simulink model "vehiclesim_mImplComplete"  (R2018a)
settings: Solver=FixedStepDiscrete  StartTime=0.0  StopTime=15  FixedStep=Ts  RelTol=1e-3  EnableMultiTasking=on
undefined symbols (not defined in the file): AL, Cd, cr1, cr2, fsw, g, i_t, Mv, p, rho_a, Rw, sigbuilder_block, Tmax, Ts, Tsi, V1, wbase
libraries: fl_lib x42, nesl_utility x16, pe_lib x5, pePwmGenerator x3, simulink x1
Description:
  | IPMSM Torque Control in an Axle-Drive EV
  | 
  | Copyright 2017 The MathWorks, Inc.
settings Model: Creator=The MathWorks, Inc.  LastModifiedBy=liamflaherty
settings SolverCC: AutoInsertRateTranBlk=on
settings DataIOCC: MaxDataPoints=510000  SignalLoggingName=logsout_pe_ipmsm_torque_control_ev_axle
settings OptimizationCC: LifeSpan=inf
settings DebuggingCC: UnderspecifiedInitializationDetection=Classic  MergeDetectMultiDrivingBlocksExec=none  SFUnexpectedBacktrackingDiag=warning  SFNoUnconditionalDefaultTransitionDiag=warning  SFExecutionAtInitializationDiag=none
settings CodeAppCC: StateflowObjectComments=on
settings GRTTargetCC: TargetLangStandard=C89/C90 (ANSI)  GeneratePreprocessorConditionals=Disable all
settings ConfigComp: CovMetricSettings=dw  CovHtmlReporting=on  CovSaveCumulativeToWorkspaceVar=on  CovSaveSingleToWorkspaceVar=on  CovExternalEMLEnable=off
settings SimscapeCC: SimscapeNormalizeSystem=off  SimscapeLogType=all  SimscapeLogSimulationStatistics=on  SimscapeLogName=simlog_pe_ipmsm_torque_control_ev_axle  SimscapeLogDataHistory=510000

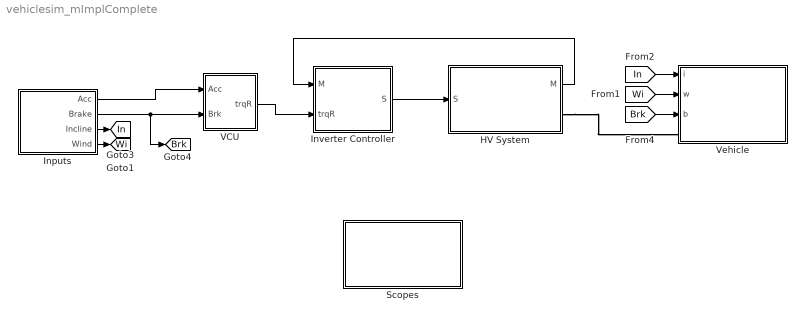
== system vehiclesim_mImplComplete ==
  HV System : Subsystem
  Inputs : Subsystem  Tag=STV Subsys  LoadFcn=sigbuilder_block('load');  StartFcn=sigbuilder_block('start');  StopFcn=sigbuilder_block('stop');  ClipboardFcn=sigbuilder_block('clipboard');  mask(Sigbuilder block){tuvar=[0:10]}
      mask help: Simulink:masks:SigbuilderBlock_MD
      mask init:
      | if ~strcmp(get_param(bdroot(gcbh),'SimulationStatus'),'stopped') tuvar = sigbuilder_block('maskInit'); end
      settings: CopyFcn=sigbuilder_block('copy');  DeleteFcn=sigbuilder_block('delete');  ModelCloseFcn=sigbuilder_block('modelClose');  PreSaveFcn=sigbuilder_block('preSave');  PauseFcn=sigbuilder_block('pause');  ContinueFcn=sigbuilder_block('continue');  NameChangeFcn=sigbuilder_block('namechange');  OpenFcn=sigbuilder_block('open',[277 144 1035 577 ]);  CloseFcn=sigbuilder_block('close');
      mask Display: plot(0, 0, 100, 100,[2, 2, 32, 32, 2], [68, 8, 8, 68, 68],[32, 2], [38, 38], [32, 19, 2],[53, 60, 44], [32, 17, 17, 2],[16, 16, 31, 31]);txt = getActiveGroup(gcbh);text(2, 100, txt,'verticalAlignment', 'top');
  Inverter Controller : Subsystem
  Scopes : Subsystem
  VCU : Subsystem
  Vehicle : Subsystem
  tag scope: Brk=global, In=global, Wi=global
  wires:
  Inputs/1(Acc) -> VCU/1(Acc)
  Inputs/3(Incline) -> [In]
  Inputs/2(Brake) -> VCU/2(Brk), [Brk]
  Inputs/4(Wind) -> [Wi]
  VCU/1(trqR) -> Inverter Controller/2(trqR)
  [In] -> Vehicle/1(i)
  [Wi] -> Vehicle/2(w)
  [Brk] -> Vehicle/3(b)
  Inverter Controller/1(S) -> HV System/1(S)
  HV System/1(M) -> Inverter Controller/1(M)
  connections:
  HV System/RConn1 -- Vehicle/LConn1

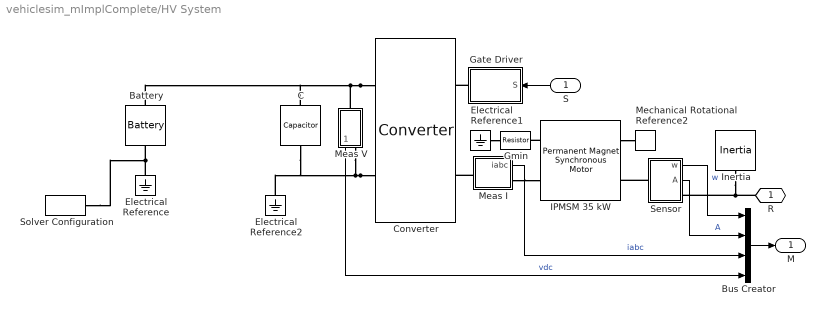
== system vehiclesim_mImplComplete/HV System ==
  S : Inport
  Battery : pe_lib/Sources/Battery  Vnom=Vnom V  R1=0.001 Ohm  prm_AH=1  AH=15000 hr*A  V1=V1 V  AH1=10000 hr*A  prm_R2=1  R2=2000 Ohm  prm_dyn=1  Rp1=0.005 Ohm  tau1=30 s  Rp2=0.005 Ohm  tau2=30 s  prm_fade=1  N_fade=100  AH_fade=45 hr*A  R1_fade=2.02 Ohm  V1_fade=10.35 V  i_specify=off  i_priority=None  i=0 A  i_nominal_specify=off  i_nominal_unit=A  i_nominal_value=1  v_specify=off  v_priority=None  v=0 V  v_nominal_specify=off  v_nominal_unit=V  v_nominal_value=1  charge_specify=on  charge_priority=High  charge=14000 hr*A  charge_nominal_specify=off  charge_nominal_unit=hr*A  charge_nominal_value=1  num_cycles_specify=off  num_cycles_priority=High  num_cycles=0  num_cycles_nominal_specify=off  num_cycles_nominal_unit=1  num_cycles_nominal_value=1  thermal_mass=30000 J/K  Tmeas=298.15 K  Vnom_T2=12 V  R1_T2=2.2 Ohm  V1_T2=11.4 V  R2_T2=2200 Ohm  Rp1_T2=0.005 Ohm  tau1_T2=30 s  Rp2_T2=0.005 Ohm  tau2_T2=30 s  Tmeas2=273.15 K  temperature_specify=off  temperature_priority=High  temperature=298.15 K  temperature_nominal_specify=off  temperature_nominal_unit=K  temperature_nominal_value=1
      settings: SourceProductName=Simscape Power Systems  SourceProductBaseCode=PS
  Bus Creator : BusCreator  Inputs=4
  C : fl_lib/Electrical/Electrical Elements/Capacitor  c=Cdc F  r=1e-6 Ohm  g=0 1/Ohm  i_specify=off  i_priority=None  i=0 A  i_nominal_specify=off  i_nominal_unit=A  i_nominal_value=1  v_specify=off  v_priority=None  v=0 V  v_nominal_specify=off  v_nominal_unit=V  v_nominal_value=1  vc_specify=off  vc_priority=High  vc=0 V  vc_nominal_specify=off  vc_nominal_unit=V  vc_nominal_value=1
      settings: SourceProductName=Foundation Library
  Converter : pe_lib/Semiconductors/Converter  device_type=3  Vf=0.8 V  Ron=0.001 Ohm  Rds=0.001 Ohm  Goff=1e-5 1/Ohm  Vth=0.5 V  Vgt=1 V  Vgt_off=-1 V  Ih=1 A  diode_param=2  diode_Vf=0.8 V  diode_Ron=0.001 Ohm  diode_Goff=1e-5 1/Ohm  diode_C=50 nF  diode_iRM=-235 A  diode_iF=300 A  diode_idot=-50 A/us  diode_trr_param=1  diode_trr_factor=3  diode_trr=15 us  diode_Qrr=1.5e+3 s*uA  snubber_type=0  Rs=0.1 Ohm  Cs=1e-7 F
      settings: SourceProductName=Simscape Power Systems  SourceProductBaseCode=PS
  Electrical Reference : fl_lib/Electrical/Electrical Elements/Electrical Reference
      settings: SourceProductName=Foundation Library
  Electrical Reference1 : fl_lib/Electrical/Electrical Elements/Electrical Reference
      settings: SourceProductName=Foundation Library
  Electrical Reference2 : fl_lib/Electrical/Electrical Elements/Electrical Reference
      settings: SourceProductName=Foundation Library
  Gate Driver : Subsystem
  Gmin : fl_lib/Electrical/Electrical Elements/Resistor  R=1e9 Ohm  i_specify=off  i_priority=High  i=0 A  i_nominal_specify=off  i_nominal_unit=A  i_nominal_value=1  v_specify=off  v_priority=High  v=0 V  v_nominal_specify=off  v_nominal_unit=V  v_nominal_value=1
      settings: SourceProductName=Foundation Library
  IPMSM 35 kW : pe_lib/Machines/Permanent Magnet Rotor/Permanent Magnet Synchronous Motor  nPolePairs=p  pmflux_param=1  pm_flux_linkage=psim Wb  torque_constant=0.18 N*m/A  back_emf_constant=0.18 V/(rad/s)  stator_param=1  Ld=Ld H  Lq=Lq H  L0=L0 H  Ls=0.0002 H  Lm=0.00002 H  Ms=0.00002 H  Rs=Rs Ohm  zero_sequence=pe.enum.park.zerosequence.exclude  J=0 kg*m^2  lam=0 N*m/(rad/s)  axes_param=1  i_d_specify=off  i_d_priority=None  i_d=0 A  i_d_nominal_specify=off  i_d_nominal_unit=A  i_d_nominal_value=1  i_q_specify=off  i_q_priority=None  i_q=0 A  i_q_nominal_specify=off  i_q_nominal_unit=A  i_q_nominal_value=1  torque_specify=off  torque_priority=None  torque=0 N*m  torque_nominal_specify=off  torque_nominal_unit=N*m  torque_nominal_value=1  angular_velocity_specify=on  angular_velocity_priority=None  angular_velocity=0 rpm  angular_velocity_nominal_specify=off  angular_velocity_nominal_unit=rpm  angular_velocity_nominal_value=1  angular_position_specify=off  angular_position_priority=None  angular_position=0 deg  angular_position_nominal_specify=off  angular_position_nominal_unit=deg  angular_position_nominal_value=1
      settings: SourceProductName=Simscape Power Systems  SourceProductBaseCode=PS
  Inertia : fl_lib/Mechanical/Rotational Elements/Inertia  inertia=Jm kg*m^2  w_specify=off  w_priority=High  w=0 rad/s  w_nominal_specify=off  w_nominal_unit=rad/s  w_nominal_value=1  t_specify=off  t_priority=None  t=0 N*m  t_nominal_specify=off  t_nominal_unit=N*m  t_nominal_value=1
      settings: SourceProductName=Foundation Library
  Meas I : Subsystem
      mask Display: %disp('iABC');
  Meas V : Subsystem
  Mechanical Rotational Reference2 : fl_lib/Mechanical/Rotational Elements/Mechanical Rotational Reference
      settings: SourceProductName=Foundation Library
  Sensor : Subsystem
  Solver Configuration : nesl_utility/Solver Configuration  PhysicalDomain=network_engine_domain  SubClassName=solver  LeftPortType=input  RightPortType=generic  Tones=[]  Harmonics=[]  SimulateNoise=off  Profile=off  UseLocalSampling=off  EnableSwitchedLinearOptims=on  FrequencyDomain=off  UseCCode=off  RelTol=0.001  AbsTol=1e-06  MinStep=1e-09  ToWorkspace=off  RevertToSquareIcSolve=off  NumHomotopyIterations=100  PhasorMode=off  PhasorModeNumHarmonics=1  DoDC=off  ResidualTolerance=1e-9  UseLocalSolver=on  LocalSolverChoice=NE_BACKWARD_EULER_ADVANCER  LocalSolverSampleTime=Ts  DoFixedCost=on  MaxNonlinIter=4  MaxModeIter=2  LinearAlgebra=Sparse  EquationFormulation=NE_TIME_EF  DelaysMemoryBudget=1024  AutomaticFiltering=on  FilteringTimeConstant=0.001
  R : PMIOPort  Side=Right
  M : Outport
  wires:
  Meas V/1(Vdc) -> Bus Creator/4  "vdc"
  Sensor/2(A) -> Bus Creator/2  "A"
  Bus Creator/1 -> M/1
  Sensor/1(w) -> Bus Creator/1  "w"
  Meas I/1(iabc) -> Bus Creator/3  "iabc"
  S/1 -> Gate Driver/1(S)
  connections:
  Converter/RConn2 -- Electrical Reference2/LConn1 -- C/RConn1 -- Meas V/RConn1
  Converter/RConn1 -- Battery/LConn1 -- C/LConn1 -- Meas V/LConn1
  Inertia/LConn1 -- R/RConn1 -- Sensor/RConn1
  IPMSM 35 kW/RConn2 -- Mechanical Rotational Reference2/LConn1
  Meas I/RConn1 -- IPMSM 35 kW/LConn1
  Gate Driver/RConn1 -- Converter/LConn1
  Meas I/LConn1 -- Converter/LConn2
  Electrical Reference1/LConn1 -- Gmin/LConn1
  Sensor/LConn1 -- IPMSM 35 kW/RConn1
  IPMSM 35 kW/LConn2 -- Gmin/RConn1
  Battery/RConn1 -- Electrical Reference/LConn1 -- Solver Configuration/RConn1

== system vehiclesim_mImplComplete/Inputs ==
  Demux : Demux  Tag=STV Demux
  FromWs : FromWorkspace  Tag=STV FromWs  VariableName=tuvar  SampleTime=0
      SigBuilderData=|
      | common.afterFinalStr = 'Extrapolate'
      | common.sampleTime = 0
      | dataSet.timeRange = [0 15]
      | dataSet.name = 'Default'
      | sbobj.Groups.Name = 'Default'
      | sbobj.Groups.Signals(1).Name = 'Acc'
      | sbobj.Groups.Signals(1).XData = [0 0.2 0.2 8 8 15]
      | sbobj.Groups.Signals(1).YData = [0 0 1 1 0 0]
      | sbobj.Groups.Signals(2).Name = 'Brake'
      | sbobj.Groups.Signals(2).XData = [0 11 11 15]
      | sbobj.Groups.Signals(2).YData = [0 0 1 1]
      | sbobj.Groups.Signals(3).Name = 'Incline'
      | sbobj.Groups.Signals(3).XData = [0 3.5 4 4.1 4.295 15]
      | sbobj.Groups.Signals(3).YData = [0 0 0 0 0 0]
      | sbobj.Groups.Signals(4).Name = 'Wind'
      | sbobj.Groups.Signals(4).XData = [0 15]
      | sbobj.Groups.Signals(4).YData = [0 0]
      | sbobj.Groups.TimeRange = [0 15]
  Acc : Outport  Tag=STV Outport
  Brake : Outport  Tag=STV Outport  Port=2
  Incline : Outport  Tag=STV Outport  Port=3
  Wind : Outport  Tag=STV Outport  Port=4
  wires:
  FromWs/1 -> Demux/1
  Demux/1 -> Acc/1
  Demux/2 -> Brake/1
  Demux/3 -> Incline/1
  Demux/4 -> Wind/1

== system vehiclesim_mImplComplete/Inverter Controller ==
  M : Inport
  trqR : Inport  Port=2
  Bus Selector : BusSelector  OutputSignals=iabc,w,A,vdc
  EM Controller : Subsystem
  S : Outport
  wires:
  M/1 -> Bus Selector/1
  trqR/1 -> EM Controller/1(trqR)
  Bus Selector/1 -> EM Controller/2(iabc_sens)  "<iabc>"
  Bus Selector/2 -> EM Controller/3(w_sens)  "<w>"
  Bus Selector/3 -> EM Controller/4(th_sens)  "<A>"
  Bus Selector/4 -> EM Controller/5(Vdc_sens)  "<vdc>"
  EM Controller/1(S) -> S/1

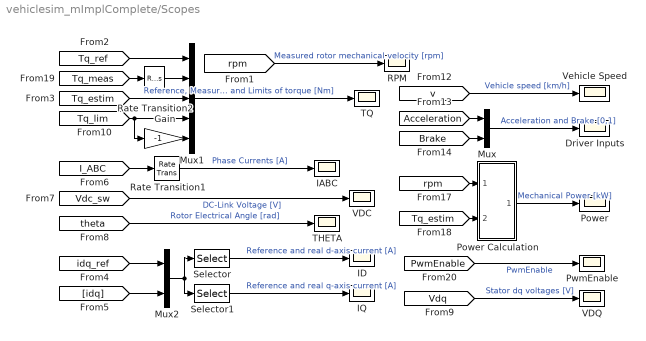
== system vehiclesim_mImplComplete/Scopes ==
  Driver Inputs : Scope
  Gain : Gain  Gain=-1
  IABC : Scope
  ID : Scope
  IQ : Scope
  Mux : Mux  Inputs=2
  Mux1 : Mux  Inputs=5
  Mux2 : Mux  Inputs=2
  Power : Scope
  Power Calculation : Subsystem
  PwmEnable : Scope
  RPM : Scope
  Rate Transition1 : RateTransition  OutPortSampleTime=1e-4
  Rate Transition2 : RateTransition
  Selector : Selector  InputPortWidth=4  IndexOptions=Index vector (dialog)  Indices=[1 3]  OutputSizes=1
  Selector1 : Selector  InputPortWidth=4  IndexOptions=Index vector (dialog)  Indices=[2 4]  OutputSizes=1
  THETA : Scope
  TQ : Scope
  VDC : Scope
  VDQ : Scope
  Vehicle Speed : Scope
  wires:
  Power Calculation/1(Power) -> Power/1  "Mechanical Power [kW]"
  Gain/1 -> Mux1/5
  [idq] -> Mux2/2
  [Tq_meas] -> Rate Transition2/1
  [Tq_estim] -> Mux1/3
  [rpm] -> Power Calculation/1(rpm)
  [Tq_estim] -> Power Calculation/2(Tq)
  [idq_ref] -> Mux2/1
  [v] -> Vehicle Speed/1  "Vehicle speed [km/h]"
  Mux1/1 -> TQ/1  "Reference, Measured, Estim and Limits of torque [Nm]"
  [Vdq] -> VDQ/1  "Stator dq voltages [V]"
  [I_ABC] -> Rate Transition1/1
  [Tq_ref] -> Mux1/1
  [Tq_lim] -> Gain/1, Mux1/4
  [PwmEnable] -> PwmEnable/1  "PwmEnable"
  Rate Transition2/1 -> Mux1/2
  [theta] -> THETA/1  "Rotor Electrical Angle [rad]"
  Selector/1 -> ID/1  "Reference and real d-axis current [A]"
  Mux2/1 -> Selector1/1, Selector/1
  Mux/1 -> Driver Inputs/1  "Acceleration and Brake [0,1]"
  Selector1/1 -> IQ/1  "Reference and real q-axis current [A]"
  [Brake] -> Mux/2
  [Acceleration] -> Mux/1
  Rate Transition1/1 -> IABC/1  "Phase Currents [A]"
  [rpm] -> RPM/1  "Measured rotor mechanical velocity [rpm]"
  [Vdc_sw] -> VDC/1  "DC-Link Voltage [V]"

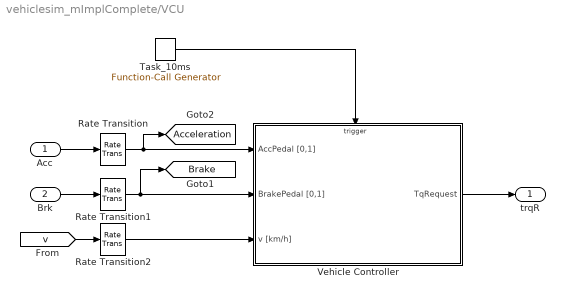
== system vehiclesim_mImplComplete/VCU ==
  Acc : Inport
  Brk : Inport  Port=2
  Rate Transition : RateTransition
  Rate Transition1 : RateTransition
  Rate Transition2 : RateTransition
  Task_10ms : simulink/Ports & Subsystems/Function-Call Generator  sample_time=0.01  numberOfIterations=1
  Vehicle Controller : Subsystem
  trqR : Outport
  tag scope: Acceleration=global, Brake=global
  wires:
  Acc/1 -> Rate Transition/1
  Task_10ms/1 -> Vehicle Controller/Trigger
  Vehicle Controller/1(TqRequest) -> trqR/1
  Brk/1 -> Rate Transition1/1
  Rate Transition/1 -> Vehicle Controller/1(AccPedal [0,1]), [Acceleration]
  Rate Transition1/1 -> [Brake], Vehicle Controller/2(BrakePedal [0,1])
  [v] -> Rate Transition2/1
  Rate Transition2/1 -> Vehicle Controller/3(v [km/h])

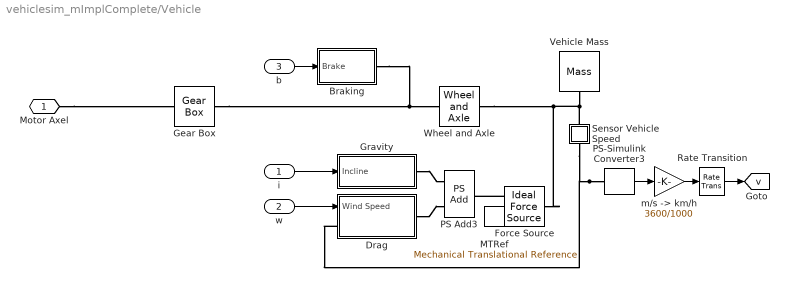
== system vehiclesim_mImplComplete/Vehicle ==
  i : Inport
  w : Inport  Port=2
  b : Inport  Port=3
  Braking : Subsystem
  Drag : Subsystem
  Force Source : fl_lib/Mechanical/Mechanical Sources/Ideal Force Source
      settings: SourceProductName=Foundation Library
  Gear Box : fl_lib/Mechanical/Mechanisms/Gear Box  ratio=i_t  t_in_specify=off  t_in_priority=None  t_in=0 N*m  t_in_nominal_specify=off  t_in_nominal_unit=N*m  t_in_nominal_value=1  t_out_specify=off  t_out_priority=None  t_out=0 N*m  t_out_nominal_specify=off  t_out_nominal_unit=N*m  t_out_nominal_value=1
      settings: SourceProductName=Foundation Library
  Gravity : Subsystem
  MTRef : fl_lib/Mechanical/Translational Elements/Mechanical Translational Reference
      settings: SourceProductName=Foundation Library
  PS Add3 : fl_lib/Physical Signals/Functions/PS Add
      settings: SourceProductName=Foundation Library
  PS-Simulink Converter3 : nesl_utility/PS-Simulink Converter  PhysicalDomain=network_engine_domain  SubClassName=ps_output  LeftPortType=input  RightPortType=output  PseudoPeriodic=off  Frequencies=[]  Unit=m/s  AffineConversion=off
  Rate Transition : RateTransition  OutPortSampleTime=1e-4
  Sensor Vehicle Speed : Subsystem
      mask Display: disp('v')
  Vehicle Mass : fl_lib/Mechanical/Translational Elements/Mass  mass=Mv kg  v_specify=off  v_priority=High  v=0 m/s  v_nominal_specify=off  v_nominal_unit=m/s  v_nominal_value=1  f_specify=off  f_priority=None  f=0 N  f_nominal_specify=off  f_nominal_unit=N  f_nominal_value=1
      settings: SourceProductName=Foundation Library
  Wheel and Axle : fl_lib/Mechanical/Mechanisms/Wheel and Axle  R=Rw m  or=1  t_specify=off  t_priority=None  t=0 N*m  t_nominal_specify=off  t_nominal_unit=N*m  t_nominal_value=1  f_specify=off  f_priority=None  f=0 N  f_nominal_specify=off  f_nominal_unit=N  f_nominal_value=1
      settings: SourceProductName=Foundation Library
  "m/s -> km/h" : Gain  Gain=3600/1000
  Motor Axel : PMIOPort  Side=Left
  tag scope: v=global
  wires:
  "m/s -> km/h"/1 -> Rate Transition/1
  Rate Transition/1 -> [v]
  b/1 -> Braking/1(Brake)
  w/1 -> Drag/1(Wind Speed)
  i/1 -> Gravity/1(Incline)
  PS-Simulink Converter3/1 -> "m/s -> km/h"/1
  connections:
  Sensor Vehicle Speed/LConn1 -- Wheel and Axle/RConn1 -- Force Source/LConn1 -- Vehicle Mass/LConn1
  Braking/RConn1 -- Wheel and Axle/LConn1 -- Gear Box/RConn1
  PS-Simulink Converter3/LConn1 -- Drag/LConn1 -- Sensor Vehicle Speed/RConn1
  Gravity/RConn1 -- PS Add3/LConn1
  MTRef/LConn1 -- Force Source/RConn2
  Drag/RConn1 -- PS Add3/LConn2
  Force Source/RConn1 -- PS Add3/RConn1
  Motor Axel/RConn1 -- Gear Box/LConn1

== system vehiclesim_mImplComplete/HV System/Gate Driver ==
  S : Inport
  Demux : Demux  Outputs=6
  Simulink-PS Converter{1..6} (6 alike) : nesl_utility/Simulink-PS Converter  PhysicalDomain=network_engine_domain  SubClassName=ps_input  LeftPortType=input  RightPortType=output  PseudoPeriodic=off  Frequencies=[]  NoiseDistribution=none  NoiseParameters=[]  Unit=1  AffineConversion=off  FilteringAndDerivatives=zero  SimscapeFilterOrder=1  InputFilterTimeConstant=0.001  UdotUserProvided=1
  Six-Pulse Gate Multiplexer : pe_lib/Semiconductors/Six-Pulse Gate Multiplexer  R=0 Ohm
      settings: SourceProductName=Simscape Power Systems  SourceProductBaseCode=PS
  G : PMIOPort  Side=Right
  wires:
  Demux/1 -> Simulink-PS Converter1/1
  S/1 -> Demux/1
  Demux/4 -> Simulink-PS Converter4/1
  Demux/2 -> Simulink-PS Converter2/1
  Demux/3 -> Simulink-PS Converter3/1
  Demux/5 -> Simulink-PS Converter5/1
  Demux/6 -> Simulink-PS Converter6/1
  connections:
  Six-Pulse Gate Multiplexer/RConn1 -- G/RConn1
  Simulink-PS Converter1/RConn1 -- Six-Pulse Gate Multiplexer/LConn1
  Simulink-PS Converter3/RConn1 -- Six-Pulse Gate Multiplexer/LConn3
  Simulink-PS Converter5/RConn1 -- Six-Pulse Gate Multiplexer/LConn5
  Simulink-PS Converter6/RConn1 -- Six-Pulse Gate Multiplexer/LConn6
  Simulink-PS Converter4/RConn1 -- Six-Pulse Gate Multiplexer/LConn4
  Simulink-PS Converter2/RConn1 -- Six-Pulse Gate Multiplexer/LConn2

== system vehiclesim_mImplComplete/HV System/Meas I ==
  Current Sensor : pe_lib/Sensors/Current Sensor
      settings: SourceProductName=Simscape Power Systems  SourceProductBaseCode=PS
  PS-Simulink Converter : nesl_utility/PS-Simulink Converter  PhysicalDomain=network_engine_domain  SubClassName=ps_output  LeftPortType=input  RightPortType=output  PseudoPeriodic=off  Frequencies=[]  Unit=A  AffineConversion=off
  1 : PMIOPort  Side=Left
  2 : PMIOPort  Port=2  Side=Right
  iabc : Outport
  tag scope: I_ABC=global
  wires:
  PS-Simulink Converter/1 -> [I_ABC], iabc/1
  connections:
  1/RConn1 -- Current Sensor/LConn1
  2/RConn1 -- Current Sensor/RConn2
  Current Sensor/RConn1 -- PS-Simulink Converter/LConn1

== system vehiclesim_mImplComplete/HV System/Meas V ==
  PS-Simulink Converter4 : nesl_utility/PS-Simulink Converter  PhysicalDomain=network_engine_domain  SubClassName=ps_output  LeftPortType=input  RightPortType=output  PseudoPeriodic=off  Frequencies=[]  Unit=V  AffineConversion=off
  Voltage Sensor : fl_lib/Electrical/Electrical Sensors/Voltage Sensor
      settings: SourceProductName=Foundation Library
  - : PMIOPort  Side=Right
  + : PMIOPort  Port=2  Side=Left
  Vdc : Outport
  wires:
  PS-Simulink Converter4/1 -> Vdc/1
  connections:
  PS-Simulink Converter4/LConn1 -- Voltage Sensor/RConn1
  Voltage Sensor/LConn1 -- +/RConn1
  Voltage Sensor/RConn2 -- -/RConn1

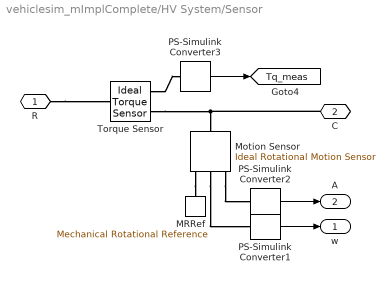
== system vehiclesim_mImplComplete/HV System/Sensor ==
  MRRef : fl_lib/Mechanical/Rotational Elements/Mechanical Rotational Reference
      settings: SourceProductName=Foundation Library
  Motion Sensor : fl_lib/Mechanical/Mechanical Sensors/Ideal Rotational Motion Sensor  offset=0 deg
      settings: SourceProductName=Foundation Library
  PS-Simulink Converter1 : nesl_utility/PS-Simulink Converter  PhysicalDomain=network_engine_domain  SubClassName=ps_output  LeftPortType=input  RightPortType=output  PseudoPeriodic=off  Frequencies=[]  Unit=rad/s  AffineConversion=off
  PS-Simulink Converter2 : nesl_utility/PS-Simulink Converter  PhysicalDomain=network_engine_domain  SubClassName=ps_output  LeftPortType=input  RightPortType=output  PseudoPeriodic=off  Frequencies=[]  Unit=rad  AffineConversion=off
  PS-Simulink Converter3 : nesl_utility/PS-Simulink Converter  PhysicalDomain=network_engine_domain  SubClassName=ps_output  LeftPortType=input  RightPortType=output  PseudoPeriodic=off  Frequencies=[]  Unit=N*m  AffineConversion=off
  Torque Sensor : fl_lib/Mechanical/Mechanical Sensors/Ideal Torque Sensor
      settings: SourceProductName=Foundation Library
  R : PMIOPort  Side=Left
  C : PMIOPort  Port=2  Side=Right
  w : Outport
  A : Outport  Port=2
  tag scope: Tq_meas=global
  wires:
  PS-Simulink Converter3/1 -> [Tq_meas]
  PS-Simulink Converter1/1 -> w/1
  PS-Simulink Converter2/1 -> A/1
  connections:
  Motion Sensor/RConn2 -- PS-Simulink Converter1/LConn1
  Motion Sensor/RConn1 -- MRRef/LConn1
  R/RConn1 -- Torque Sensor/LConn1
  Torque Sensor/RConn1 -- C/RConn1 -- Motion Sensor/LConn1
  Torque Sensor/RConn2 -- PS-Simulink Converter3/LConn1
  Motion Sensor/RConn3 -- PS-Simulink Converter2/LConn1

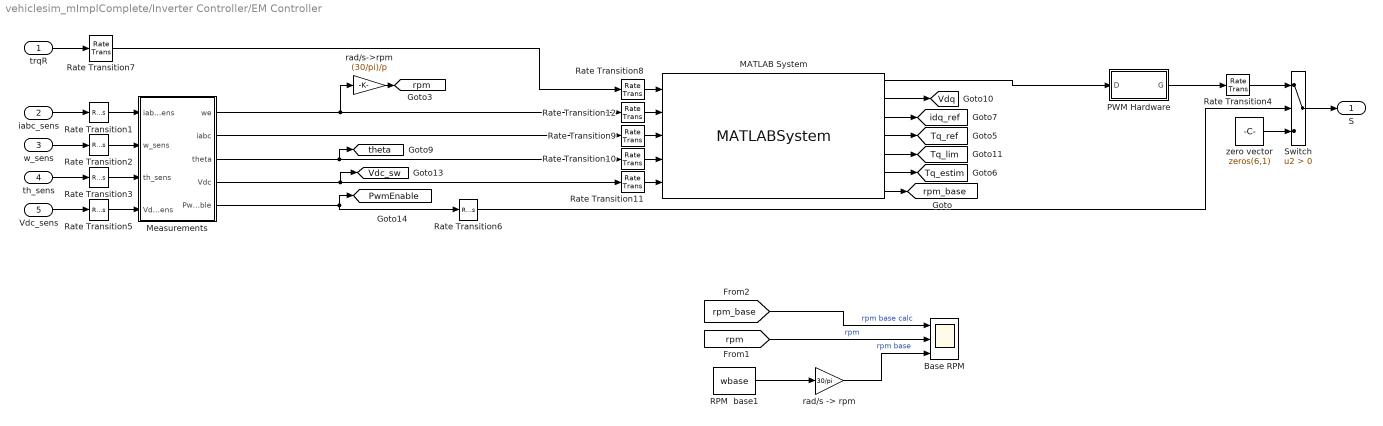
== system vehiclesim_mImplComplete/Inverter Controller/EM Controller ==
  trqR : Inport
  iabc_sens : Inport  Port=2
  w_sens : Inport  Port=3
  th_sens : Inport  Port=4
  Vdc_sens : Inport  Port=5
  Base RPM : Scope  NumInputPorts=3
  MATLAB System : MATLABSystem  System=FieldOrientedControl  T=Tsi  Vnom=Vnom  Pmax=Pmax  Tmax=Tmax  Imax=Imax  p=p  psim=psim  Rs=Rs  Ld=Ld  Lq=Lq  wBase=wbase  Kp_id=Kp_id  Ki_id=Ki_id  AntiWindUpD=1  Kp_iq=Kp_iq  Ki_iq=Ki_iq  AntiWindUpQ=1  SimulateUsing=Code generation
      mask Type: FieldOrientedControl
      mask Display:
      | disp('FieldOrientedControl');
      | port_label('input',1,'TqRef');
      | port_label('input',2,'we');
      | port_label('input',3,'iabc');
      | port_label('input',4,'theta_e');
      | port_label('input',5,'Vdc');
      | port_label('output',1,'Dabc');
      | port_label('output',2,'Vdq');
      | port_label('output',3,'idqRef');
      | port_label('output',4,'TqRefSat');
      | port_label('output',5,'TqLim');
      | port_label('output',6,'TqEst');
      | port_label('output',7,'rpm_base');
  Measurements : Subsystem
  PWM Hardware : Subsystem
  RPM  base1 : Constant  Value=wbase
  Rate Transition{1..3,5,7..12} (10 alike) : RateTransition  OutPortSampleTime=Tsi
  Rate Transition4 : RateTransition
  Rate Transition6 : RateTransition
  Switch : Switch  Criteria=u2 > Threshold
  "rad/s -> rpm" : Gain  Gain=30/pi
  rad/s->rpm : Gain  Gain=(30/pi)/p
  zero vector : Constant  Value=zeros(6,1)
  S : Outport
  tag scope: PwmEnable=global, Tq_estim=global, Tq_lim=global, Tq_ref=global, Vdc_sw=global, Vdq=global, idq_ref=global, rpm=global, rpm_base=global, theta=global
  wires:
  Measurements/5(PwmEnable) -> [PwmEnable], Rate Transition6/1
  Rate Transition7/1 -> Rate Transition8/1
  Rate Transition3/1 -> Measurements/3(th_sens)
  Rate Transition6/1 -> Switch/2
  trqR/1 -> Rate Transition7/1
  Vdc_sens/1 -> Rate Transition5/1
  Measurements/4(Vdc) -> [Vdc_sw], Rate Transition11/1
  Measurements/1(we) -> Rate Transition12/1, rad/s->rpm/1
  Rate Transition5/1 -> Measurements/4(Vdc_sens)
  rad/s->rpm/1 -> [rpm]
  Measurements/3(theta) -> Rate Transition10/1, [theta]
  iabc_sens/1 -> Rate Transition1/1
  th_sens/1 -> Rate Transition3/1
  Rate Transition2/1 -> Measurements/2(w_sens)
  Rate Transition4/1 -> Switch/1
  Switch/1 -> S/1
  w_sens/1 -> Rate Transition2/1
  Rate Transition1/1 -> Measurements/1(iabc_sens)
  zero vector/1 -> Switch/3
  Measurements/2(iabc) -> Rate Transition9/1
  PWM Hardware/1(G) -> Rate Transition4/1
  Rate Transition11/1 -> MATLAB System/5
  Rate Transition10/1 -> MATLAB System/4
  MATLAB System/1 -> PWM Hardware/1(D)
  Rate Transition8/1 -> MATLAB System/1
  MATLAB System/2 -> [Vdq]
  Rate Transition9/1 -> MATLAB System/3
  Rate Transition12/1 -> MATLAB System/2
  MATLAB System/3 -> [idq_ref]
  MATLAB System/4 -> [Tq_ref]
  MATLAB System/5 -> [Tq_lim]
  MATLAB System/6 -> [Tq_estim]
  [rpm] -> Base RPM/2  "rpm"
  [rpm_base] -> Base RPM/1  "rpm base calc"
  "rad/s -> rpm"/1 -> Base RPM/3  "rpm base"
  RPM  base1/1 -> "rad/s -> rpm"/1
  MATLAB System/7 -> [rpm_base]

== system vehiclesim_mImplComplete/Scopes/Power Calculation ==
  rpm : Inport
  Tq : Inport  Port=2
  Gain3 : Gain  Gain=pi/30
  Gain4 : Gain  Gain=1/1000
  Product2 : Product
  Power : Outport
  wires:
  rpm/1 -> Gain3/1
  Gain4/1 -> Power/1
  Product2/1 -> Gain4/1
  Tq/1 -> Product2/2
  Gain3/1 -> Product2/1

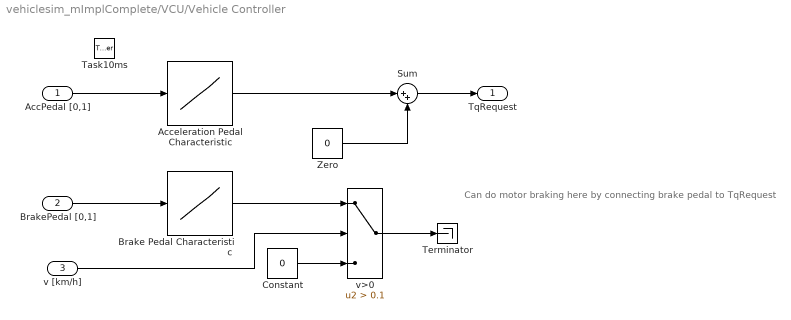
== system vehiclesim_mImplComplete/VCU/Vehicle Controller ==
  note: Can do motor braking here by connecting brake pedal to TqRequest
  AccPedal [0,1] : Inport
  BrakePedal [0,1] : Inport  Port=2
  v [km/h] : Inport  Port=3
  Task10ms : TriggerPort  TriggerType=function-call  VariantControl=Variant  PortDimensions=1
  Acceleration Pedal Characteristic : Lookup_n-D  NumberOfTableDimensions=1  BreakpointsForDimension1=0:0.1:1  Table=[0 0.04 0.07 0.1 0.16 0.2 0.3 0.4 0.6 0.8 1]*Tmax  InternalRulePriority=Speed  RndMeth=Simplest  InputSameDT=on
  Brake Pedal Characteristic : Lookup_n-D  NumberOfTableDimensions=1  BreakpointsForDimension1=[0 0.03 0.04 0.3 0.4 0.5 0.6 0.7 0.8 0.9 1]  Table=[0 0 0.04 0.05 0.06 0.2 0.25 0.4 0.6 0.8 1]*(-Tmax)  InternalRulePriority=Speed  RndMeth=Simplest  InputSameDT=on
  Constant : Constant  Value=0  SampleTime=-1
  Sum : Sum  Inputs=|++
  Terminator : Terminator
  Zero : Constant  Value=0
  v>0 : Switch  Criteria=u2 > Threshold  Threshold=0.1
  TqRequest : Outport
  wires:
  AccPedal [0,1]/1 -> Acceleration Pedal Characteristic/1
  BrakePedal [0,1]/1 -> Brake Pedal Characteristic/1
  Acceleration Pedal Characteristic/1 -> Sum/1
  Sum/1 -> TqRequest/1
  Brake Pedal Characteristic/1 -> v>0/1
  Constant/1 -> v>0/3
  v [km/h]/1 -> v>0/2
  v>0/1 -> Terminator/1
  Zero/1 -> Sum/2

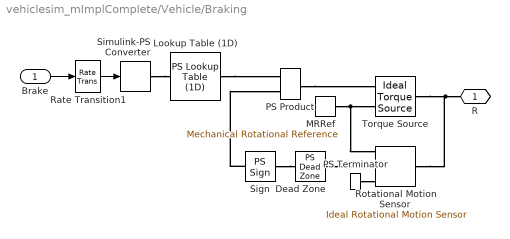
== system vehiclesim_mImplComplete/Vehicle/Braking ==
  Brake : Inport
  Dead Zone : fl_lib/Physical Signals/Nonlinear Operators/PS Dead Zone  upper_limit=0.1  lower_limit=-0.001
      settings: SourceProductName=Foundation Library
  Lookup Table (1D) : fl_lib/Physical Signals/Lookup Tables/PS Lookup Table (1D)  x=[0 0.03 0.04 0.3 0.4 0.5 0.6 0.7 0.8 0.9 1]  f=[0 0 0.04 0.05 0.06 0.2 0.25 0.4 0.6 0.8 1]*(-Tmax)*i_t  interp_method=1  extrap_method=1
      settings: SourceProductName=Foundation Library
  MRRef : fl_lib/Mechanical/Rotational Elements/Mechanical Rotational Reference
      settings: SourceProductName=Foundation Library
  PS Product : fl_lib/Physical Signals/Functions/PS Product
      settings: SourceProductName=Foundation Library
  PS Terminator : fl_lib/Physical Signals/Sinks/PS Terminator
      settings: SourceProductName=Foundation Library
  Rate Transition1 : RateTransition
  Rotational Motion Sensor : fl_lib/Mechanical/Mechanical Sensors/Ideal Rotational Motion Sensor  offset=0 rad
      settings: SourceProductName=Foundation Library
  Sign : fl_lib/Physical Signals/Nonlinear Operators/PS Sign
      settings: SourceProductName=Foundation Library
  Simulink-PS Converter : nesl_utility/Simulink-PS Converter  PhysicalDomain=network_engine_domain  SubClassName=ps_input  LeftPortType=input  RightPortType=output  PseudoPeriodic=off  Frequencies=[]  NoiseDistribution=none  NoiseParameters=[]  Unit=1  AffineConversion=off  FilteringAndDerivatives=zero  SimscapeFilterOrder=1  InputFilterTimeConstant=0.001  UdotUserProvided=1
  Torque Source : fl_lib/Mechanical/Mechanical Sources/Ideal Torque Source
      settings: SourceProductName=Foundation Library
  R : PMIOPort  Side=Right
  wires:
  Brake/1 -> Rate Transition1/1
  Rate Transition1/1 -> Simulink-PS Converter/1
  connections:
  Torque Source/LConn1 -- Rotational Motion Sensor/LConn1 -- R/RConn1
  PS Product/RConn1 -- Torque Source/RConn1
  MRRef/LConn1 -- Rotational Motion Sensor/RConn1 -- Torque Source/RConn2
  PS Terminator/LConn1 -- Rotational Motion Sensor/RConn3
  Dead Zone/LConn1 -- Rotational Motion Sensor/RConn2
  Lookup Table (1D)/RConn1 -- PS Product/LConn1
  Sign/RConn1 -- PS Product/LConn2
  Simulink-PS Converter/RConn1 -- Lookup Table (1D)/LConn1
  Sign/LConn1 -- Dead Zone/RConn1

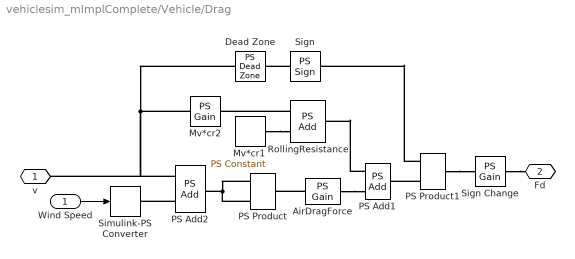
== system vehiclesim_mImplComplete/Vehicle/Drag ==
  Wind Speed : Inport
  AirDragForce : fl_lib/Physical Signals/Functions/PS Gain  gain=0.5*rho_a*AL*Cd
      settings: SourceProductName=Foundation Library
  Dead Zone : fl_lib/Physical Signals/Nonlinear Operators/PS Dead Zone  upper_limit=0.1  lower_limit=-0.001
      settings: SourceProductName=Foundation Library
  Mv*cr1 : fl_lib/Physical Signals/Sources/PS Constant  constant=Mv*cr1
      settings: SourceProductName=Foundation Library
  Mv*cr2 : fl_lib/Physical Signals/Functions/PS Gain  gain=Mv*cr2
      settings: SourceProductName=Foundation Library
  PS Add1 : fl_lib/Physical Signals/Functions/PS Add
      settings: SourceProductName=Foundation Library
  PS Add2 : fl_lib/Physical Signals/Functions/PS Add
      settings: SourceProductName=Foundation Library
  PS Product : fl_lib/Physical Signals/Functions/PS Product
      settings: SourceProductName=Foundation Library
  PS Product1 : fl_lib/Physical Signals/Functions/PS Product
      settings: SourceProductName=Foundation Library
  RollingResistance : fl_lib/Physical Signals/Functions/PS Add
      settings: SourceProductName=Foundation Library
  Sign : fl_lib/Physical Signals/Nonlinear Operators/PS Sign
      settings: SourceProductName=Foundation Library
  Sign Change : fl_lib/Physical Signals/Functions/PS Gain  gain=-1
      settings: SourceProductName=Foundation Library
  Simulink-PS Converter : nesl_utility/Simulink-PS Converter  PhysicalDomain=network_engine_domain  SubClassName=ps_input  LeftPortType=input  RightPortType=output  PseudoPeriodic=off  Frequencies=[]  NoiseDistribution=none  NoiseParameters=[]  Unit=m/s  AffineConversion=off  FilteringAndDerivatives=zero  SimscapeFilterOrder=1  InputFilterTimeConstant=0.001  UdotUserProvided=1
  v : PMIOPort  Side=Left
  Fd : PMIOPort  Port=2  Side=Right
  wires:
  Wind Speed/1 -> Simulink-PS Converter/1
  connections:
  AirDragForce/RConn1 -- PS Add1/LConn2
  PS Product1/LConn2 -- PS Add1/RConn1
  PS Add2/LConn2 -- Simulink-PS Converter/RConn1
  PS Product/LConn1 -- PS Product/LConn2 -- PS Add2/RConn1
  PS Product1/LConn1 -- Sign/RConn1
  Sign Change/RConn1 -- Fd/RConn1
  AirDragForce/LConn1 -- PS Product/RConn1
  PS Add1/LConn1 -- RollingResistance/RConn1
  Mv*cr1/RConn1 -- RollingResistance/LConn2
  Sign/LConn1 -- Dead Zone/RConn1
  RollingResistance/LConn1 -- Mv*cr2/RConn1
  PS Product1/RConn1 -- Sign Change/LConn1
  Dead Zone/LConn1 -- PS Add2/LConn1 -- v/RConn1 -- Mv*cr2/LConn1

== system vehiclesim_mImplComplete/Vehicle/Gravity ==
  Incline : Inport
  GravitationalForce : fl_lib/Physical Signals/Functions/PS Gain  gain=-1
      settings: SourceProductName=Foundation Library
  Mv*g : fl_lib/Physical Signals/Functions/PS Gain  gain=Mv*g
      settings: SourceProductName=Foundation Library
  Simulink-PS Converter1 : nesl_utility/Simulink-PS Converter  PhysicalDomain=network_engine_domain  SubClassName=ps_input  LeftPortType=input  RightPortType=output  PseudoPeriodic=off  Frequencies=[]  NoiseDistribution=none  NoiseParameters=[]  Unit=rad  AffineConversion=off  FilteringAndDerivatives=zero  SimscapeFilterOrder=1  InputFilterTimeConstant=0.001  UdotUserProvided=1
  deg->rad : Gain  Gain=pi/180
  sin : fl_lib/Physical Signals/Functions/PS Math Function  fcn_choice=1
      settings: SourceProductName=Foundation Library
  Fg : PMIOPort  Side=Right
  wires:
  Incline/1 -> deg->rad/1
  deg->rad/1 -> Simulink-PS Converter1/1
  connections:
  Simulink-PS Converter1/RConn1 -- sin/LConn1
  Mv*g/LConn1 -- sin/RConn1
  Mv*g/RConn1 -- GravitationalForce/LConn1
  GravitationalForce/RConn1 -- Fg/RConn1

== system vehiclesim_mImplComplete/Vehicle/Sensor Vehicle Speed ==
  MTRef15 : fl_lib/Mechanical/Translational Elements/Mechanical Translational Reference
      settings: SourceProductName=Foundation Library
  PS Terminator : fl_lib/Physical Signals/Sinks/PS Terminator
      settings: SourceProductName=Foundation Library
  Translational Motion Sensor : fl_lib/Mechanical/Mechanical Sensors/Ideal Translational Motion Sensor  offset=0 m
      settings: SourceProductName=Foundation Library
  Conn1 : PMIOPort  Side=Left
  Conn2 : PMIOPort  Port=2  Side=Right
  connections:
  Translational Motion Sensor/LConn1 -- Conn1/RConn1
  Translational Motion Sensor/RConn1 -- MTRef15/LConn1
  Translational Motion Sensor/RConn2 -- Conn2/RConn1
  Translational Motion Sensor/RConn3 -- PS Terminator/LConn1

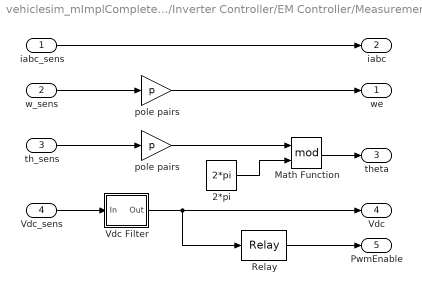
== system vehiclesim_mImplComplete/Inverter Controller/EM Controller/Measurements ==
  iabc_sens : Inport
  w_sens : Inport  Port=2
  th_sens : Inport  Port=3
  Vdc_sens : Inport  Port=4
  2*pi : Constant  Value=2*pi  SampleTime=Tsi
  Math Function : Math  Operator=mod  SaturateOnIntegerOverflow=on
  Relay : Relay  OnSwitchValue=V1/2  OffSwitchValue=V1/4
  Vdc Filter : Subsystem  mask(Discrete first-order filter (Low-pass)){T=0.01, Ts=Tsi}
      mask prompts: T "Time constant (s):"; Ts "Sample time (s):"
      mask help: This block implements a discrete low-pass filter. To calculate the coefficients, the block discretises a continuous low-pass filter using the Tustin method.
      mask init:
      | num = [ Ts/(2*T + Ts), Ts/(2*T + Ts)];
      | den = [ 1, -(2*T - Ts)/(2*T + Ts)];
  pole pairs : Gain  Gain=p
  "pole pairs " : Gain  Gain=p
  we : Outport
  iabc : Outport  Port=2
  theta : Outport  Port=3
  Vdc : Outport  Port=4
  PwmEnable : Outport  Port=5
  wires:
  pole pairs/1 -> we/1
  th_sens/1 -> "pole pairs "/1
  w_sens/1 -> pole pairs/1
  iabc_sens/1 -> iabc/1
  2*pi/1 -> Math Function/2
  Math Function/1 -> theta/1
  "pole pairs "/1 -> Math Function/1
  Vdc_sens/1 -> Vdc Filter/1(In)
  Relay/1 -> PwmEnable/1
  Vdc Filter/1(Out) -> Relay/1, Vdc/1

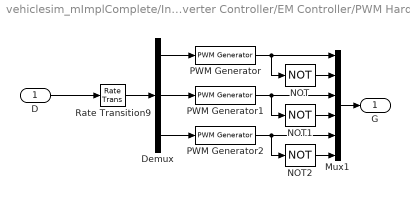
== system vehiclesim_mImplComplete/Inverter Controller/EM Controller/PWM Hardware ==
  D : Inport
  Demux : Demux  Outputs=3
  Mux1 : Mux  Inputs=6
  NOT : Logic  Operator=NOT  IconShape=distinctive  AllPortsSameDT=off  OutDataTypeStr=boolean
  NOT1 : Logic  Operator=NOT  IconShape=distinctive  AllPortsSameDT=off  OutDataTypeStr=boolean
  NOT2 : Logic  Operator=NOT  IconShape=distinctive  AllPortsSameDT=off  OutDataTypeStr=boolean
  PWM Generator : pePwmGenerator/PWM Generator  CarrCount=Up  Tper=1/fsw  Ts=Ts
  PWM Generator1 : pePwmGenerator/PWM Generator  CarrCount=Up  Tper=1/fsw  Ts=Ts
  PWM Generator2 : pePwmGenerator/PWM Generator  CarrCount=Up  Tper=1/fsw  Ts=Ts
  Rate Transition9 : RateTransition
  G : Outport
  wires:
  PWM Generator/1 -> NOT/1, Mux1/1
  Demux/1 -> PWM Generator/1
  NOT1/1 -> Mux1/4
  PWM Generator1/1 -> Mux1/3, NOT1/1
  NOT2/1 -> Mux1/6
  NOT/1 -> Mux1/2
  PWM Generator2/1 -> Mux1/5, NOT2/1
  Demux/2 -> PWM Generator1/1
  Demux/3 -> PWM Generator2/1
  Mux1/1 -> G/1
  D/1 -> Rate Transition9/1
  Rate Transition9/1 -> Demux/1

== system vehiclesim_mImplComplete/Inverter Controller/EM Controller/Measurements/Vdc Filter ==
  In : Inport
  Discrete Transfer Fcn : DiscreteTransferFcn  Numerator=num  Denominator=den
  Out : Outport
  wires:
  In/1 -> Discrete Transfer Fcn/1
  Discrete Transfer Fcn/1 -> Out/1
